simulink model "DemonstratorSimscape"  (R2020b)
settings: Solver=ode113  StartTime=0.0  StopTime=t_stop*0+20  FixedStep=1e-4
values from neighbouring files (symbols this model uses):
  brkD = 0    [main.m]
  brkI = 1e4    (= 10000)    [main.m]
  brkP = 1e5    (= 100000)    [main.m]
  d_drm = 0.5*d_drum    [main.m]
  d_shm = 0.4*d_sheave    [main.m]
  DeltaCable0 = 0    [main.m]
  Droop_scaling = 0    [main.m]
  eta_sh = 0.015    [main.m]
  filt_NUM = ones(1,200)*0.005    [main.m]
  g = 9.80665    [main.m]
  Iw = 0.5*(W.i + M.in*GB.r^2)    [main.m]
  Kp_mul = 0.3    [main.m]
  Lc0 = abs((T.ph-L.height-P.d-L.z0)*0.001)    [main.m]
  Ls1 = ((T.ph-0.5*W.pd)/1000)    [main.m]
  Ls2 = ((0.5*(T.s2+P.d)-2*P.d)/1000)    [main.m]
  M = 50e3    (= 50000)    [calcGrav.m]
  phi0_drm = -90    [main.m]
  phi0_shm = -90    [main.m]
  r_sheave = P.d*0.5    [main.m]
  s = tf('s')    [calcGrav.m]
  tau_brk = 0.001    [main.m]
  tau_em = 60e-3    (= 0.06)    [calcGrav.m]    (also in main.m)
  tau_m = tau_w/GB.r    [main.m]
  Tmax = 400e3    (= 400000)    [main.m]
  Tn_mul = 10    [main.m]
  x_drm = 0.7*r_drum    [main.m]
  x_shm = 0.7*r_sheave    [main.m]
  z0 = 0    [calcGrav.m]    (also in main.m = L.z0-P.d*0.5-P.d-P.d-L.height-T.h1-T.h2-32)
undefined symbols (not defined in the file or in its folder): C, CA, Controller_sampleTime, DiscIntNeverNeededParam, GB, L, P, Part, T, VFD_acceleration_model_factor, VFD_Adapt_factor_lower_p1458, VFD_Adapt_factor_upper_p1459, VFD_Curr_limit_var_p0641, VFD_Current_limit_p0640, VFD_Id_setp_total_r1624, VFD_Iq, VFD_Kp_n_basic_p1460, VFD_M, VFD_M_accel_T_smooth_p1517, VFD_M_lim_var_fixS_src_p1551, VFD_M_max_lower_p1521, VFD_M_max_lower_scal_p1525, VFD_M_max_up_mot_scal_p1524, VFD_M_max_upper_p1520, VFD_n_act_T_smooth_p1442, VFD_n_ctr_Kp_n_up_scal_p1461, VFD_n_ctr_Tn_n_up_sca_p1463, VFD_n_ctrl_adapt_Kp_lower_p1456, VFD_n_ctrl_adapt_Kp_upper_p1457, VFD_n_ctrl_Adpt_sig_Kp_p1455, VFD_n_ctrl_Kp_scal_p1466, VFD_n_ctrl_n_lower_p1464, VFD_n_ctrl_n_upper_p1465, VFD_n_ctrl_Tn_n_lower_p1462, VFD_n_limit_neg_p1086, VFD_n_limit_pos_p1083, VFD_n_limit_setp_p1063, VFD_n_max_p1082, VFD_n_set_filt_1_T_p1416, VFD_P_max_gen_p1531, VFD_P_max_mot_p1530, VFD_PU_I_outp_max_r0289, VFD_RFG_ramp_down_time_p1121, VFD_RFG_ramp_up_time_p1120, VFD_RFG_t_RD_scal_p1139, VFD_RFG_t_RU_scal_p1138, VSD, W, X, Y, Z
libraries: sm_lib x248, nesl_utility x128, simulink x49, pid_lib x4, cstblocks x2, simulink_extras x2
(part 2 of 10)

== system DemonstratorSimscape/EM System/Winch Left (yellow) ==
  theta winch (deg) : Inport
  Rigid Transform : sm_lib/Frames and Transforms/Rigid Transform  TranslationMethod=None  TranslationStandardOffset=0  TranslationLengthUnit=m  TranslationStandardAxis=+Z  TranslationCartesianOffset=[0 0 0]  TranslationROffset=0  TranslationROffsetUnits=m  TranslationZOffset=0  TranslationZOffsetUnits=m  TranslationThetaOffset=0  TranslationThetaOffsetUnits=deg  RotationMethod=StandardAxis  RotationAngleUnits=deg  RotationStandardAxis=+X  RotationAngle=90  RotationArbitraryAxis=[0 0 1]  FollAlignAxisA=+X  BaseAlignAxisA=+Y  FollAlignAxisB=+Y  BaseAlignAxisB=+Z  RotationSequenceAxes=FollowerAxes  RotationSequence=XYX  RotationSequenceAngles=[0 0 0]  RotationSequenceAnglesUnits=deg  RotationMatrix=[1 0 0; 0 1 0; 0 0 1]
  Rigid Transform1 : sm_lib/Frames and Transforms/Rigid Transform  TranslationMethod=StandardAxis  TranslationStandardOffset=1.2*W.w/2  TranslationLengthUnit=mm  TranslationStandardAxis=-Z  TranslationCartesianOffset=[0 0 0]  TranslationROffset=0  TranslationROffsetUnits=m  TranslationZOffset=0  TranslationZOffsetUnits=m  TranslationThetaOffset=0  TranslationThetaOffsetUnits=deg  RotationMethod=None  RotationAngleUnits=deg  RotationStandardAxis=+Z  RotationAngle=0.0  RotationArbitraryAxis=[0 0 1]  FollAlignAxisA=+X  BaseAlignAxisA=+Y  FollAlignAxisB=+Y  BaseAlignAxisB=+Z  RotationSequenceAxes=FollowerAxes  RotationSequence=XYX  RotationSequenceAngles=[0 0 0]  RotationSequenceAnglesUnits=deg  RotationMatrix=[1 0 0; 0 1 0; 0 0 1]
  Rigid Transform2 : sm_lib/Frames and Transforms/Rigid Transform  TranslationMethod=None  TranslationStandardOffset=0  TranslationLengthUnit=m  TranslationStandardAxis=+Z  TranslationCartesianOffset=[0 0 0]  TranslationROffset=0  TranslationROffsetUnits=m  TranslationZOffset=0  TranslationZOffsetUnits=m  TranslationThetaOffset=0  TranslationThetaOffsetUnits=deg  RotationMethod=StandardAxis  RotationAngleUnits=deg  RotationStandardAxis=+Z  RotationAngle=0  RotationArbitraryAxis=[0 0 1]  FollAlignAxisA=+X  BaseAlignAxisA=+Y  FollAlignAxisB=+Y  BaseAlignAxisB=+Z  RotationSequenceAxes=FollowerAxes  RotationSequence=XYX  RotationSequenceAngles=[0 0 0]  RotationSequenceAnglesUnits=deg  RotationMatrix=[1 0 0; 0 1 0; 0 0 1]
  Transform Winch Axis1 : sm_lib/Frames and Transforms/Rigid Transform  TranslationMethod=None  TranslationStandardOffset=0  TranslationLengthUnit=m  TranslationStandardAxis=+Z  TranslationCartesianOffset=[0 0 0]  TranslationROffset=0  TranslationROffsetUnits=m  TranslationZOffset=0  TranslationZOffsetUnits=m  TranslationThetaOffset=0  TranslationThetaOffsetUnits=deg  RotationMethod=StandardAxis  RotationAngleUnits=deg  RotationStandardAxis=+Y  RotationAngle=180  RotationArbitraryAxis=[0 0 1]  FollAlignAxisA=+X  BaseAlignAxisA=+Y  FollAlignAxisB=+Y  BaseAlignAxisB=+Z  RotationSequenceAxes=FollowerAxes  RotationSequence=XYX  RotationSequenceAngles=[0 0 0]  RotationSequenceAnglesUnits=deg  RotationMatrix=[1 0 0; 0 1 0; 0 0 1]
  Variable Winch Inertia : Subsystem
  Winch1 : sm_lib/Body Elements/Cylindrical Solid  GraphicAmbientColor=[0.15 0.15 0.15 1.0]  BasedOnType=Mass  CenterOfMass=[0 0 W.w*0.5]  CenterOfMassUnits=m  GraphicDiffuseColor=[1.0 1.0 1.0]  CylinderLength=W.w  CylinderLengthUnits=mm  CylinderRadius=W.d*0.5  CylinderRadiusUnits=mm  Density=0  DensityUnits=kg/m^3  DoExposeReferenceFrame=off  GraphicEmissiveColor=[0.0 0.0 0.0 1.0]  ExportEntireGeometry=off  SerializedFrames=<Frames><Frame><Id>Frame1</Id><Value><Name>F1</Name><Origin><Source>ReferenceFrame</Source><FeatureName></FeatureName></Origin><PrimaryAxis><DefinedDirection>+Z</DefinedDirection><Source>ReferenceFrame</Source><SourceDirection>-Y</SourceDirection><FeatureName></FeatureName></PrimaryAxis><SecondaryAxis><DefinedDirection>+X</DefinedDirection><Source>ReferenceFrame</Source><SourceDirection>+X</SourceDirection><FeatureName></FeatureName></SecondaryAxis></Value></Frame></Frames>  MarkerShape=Frame  MarkerSize=10  GraphicType=FromGeometry  InertiaType=CalculateFromGeometry  Mass=W.mass  MassUnits=kg  MomentsOfInertia=[1 1 1]*Iw  MomentsOfInertiaUnits=kg*m^2  GraphicOpacity=1.0  ProductsOfInertia=[0 0 0]  ProductsOfInertiaUnits=kg*m^2  GraphicShininess=10  GraphicSpecularColor=[0.8 0.8 0.8]  GraphicVisPropType=SimpleVisualProperties
  tags : Subsystem  mask{phi0=phi0_drm, s=1}
      mask prompts: phi0 "angle (deg)"; s "direction (1 | -1)"
  W : PMIOPort  Side=Right
  F : PMIOPort  Port=2  Side=Left
  r_winch (mm) : Outport  VectorParamsAs1DForOutWhenUnconnected=off
  wires:
  theta winch (deg)/1 -> Variable Winch Inertia/1(WinchAngle (deg))
  Variable Winch Inertia/2(WinchRadius (mm)) -> r_winch (mm)/1
  connections:
  W/RConn1 -- Rigid Transform2/RConn1 -- Transform Winch Axis1/RConn1
  Winch1/LConn1 -- Rigid Transform/LConn1 -- Variable Winch Inertia/RConn1
  Rigid Transform/RConn1 -- Rigid Transform2/LConn1
  Transform Winch Axis1/LConn1 -- Rigid Transform1/LConn1 -- F/RConn1
  tags/LConn1 -- Rigid Transform1/RConn1

== system DemonstratorSimscape/EM System/Winch Right (blue) ==
  theta winch (deg) : Inport
  Rigid Transform : sm_lib/Frames and Transforms/Rigid Transform  TranslationMethod=None  TranslationStandardOffset=0  TranslationLengthUnit=m  TranslationStandardAxis=+Z  TranslationCartesianOffset=[0 0 0]  TranslationROffset=0  TranslationROffsetUnits=m  TranslationZOffset=0  TranslationZOffsetUnits=m  TranslationThetaOffset=0  TranslationThetaOffsetUnits=deg  RotationMethod=StandardAxis  RotationAngleUnits=deg  RotationStandardAxis=+X  RotationAngle=90  RotationArbitraryAxis=[0 0 1]  FollAlignAxisA=+X  BaseAlignAxisA=+Y  FollAlignAxisB=+Y  BaseAlignAxisB=+Z  RotationSequenceAxes=FollowerAxes  RotationSequence=XYX  RotationSequenceAngles=[0 0 0]  RotationSequenceAnglesUnits=deg  RotationMatrix=[1 0 0; 0 1 0; 0 0 1]
  Rigid Transform1 : sm_lib/Frames and Transforms/Rigid Transform  TranslationMethod=StandardAxis  TranslationStandardOffset=1.05*W.w/2  TranslationLengthUnit=mm  TranslationStandardAxis=+Z  TranslationCartesianOffset=[0 0 0]  TranslationROffset=0  TranslationROffsetUnits=m  TranslationZOffset=0  TranslationZOffsetUnits=m  TranslationThetaOffset=0  TranslationThetaOffsetUnits=deg  RotationMethod=None  RotationAngleUnits=deg  RotationStandardAxis=+Z  RotationAngle=0.0  RotationArbitraryAxis=[0 0 1]  FollAlignAxisA=+X  BaseAlignAxisA=+Y  FollAlignAxisB=+Y  BaseAlignAxisB=+Z  RotationSequenceAxes=FollowerAxes  RotationSequence=XYX  RotationSequenceAngles=[0 0 0]  RotationSequenceAnglesUnits=deg  RotationMatrix=[1 0 0; 0 1 0; 0 0 1]
  Variable Winch Inertia : Subsystem
  Winch2 : sm_lib/Body Elements/Cylindrical Solid  GraphicAmbientColor=[0.15 0.15 0.15 1.0]  BasedOnType=Mass  CenterOfMass=[0 0 W.w*0.5]  CenterOfMassUnits=m  GraphicDiffuseColor=[1.0 1.0 1.0]  CylinderLength=W.w  CylinderLengthUnits=mm  CylinderRadius=W.d*0.5  CylinderRadiusUnits=mm  Density=0  DensityUnits=kg/m^3  DoExposeReferenceFrame=off  GraphicEmissiveColor=[0.0 0.0 0.0 1.0]  ExportEntireGeometry=off  SerializedFrames=<Frames><Frame><Id>Frame1</Id><Value><Name>F1</Name><Origin><Source>ReferenceFrame</Source><FeatureName></FeatureName></Origin><PrimaryAxis><DefinedDirection>+Z</DefinedDirection><Source>ReferenceFrame</Source><SourceDirection>-Y</SourceDirection><FeatureName></FeatureName></PrimaryAxis><SecondaryAxis><DefinedDirection>+X</DefinedDirection><Source>ReferenceFrame</Source><SourceDirection>+X</SourceDirection><FeatureName></FeatureName></SecondaryAxis></Value></Frame></Frames>  MarkerShape=Frame  MarkerSize=10  GraphicType=FromGeometry  InertiaType=CalculateFromGeometry  Mass=W.mass  MassUnits=kg  MomentsOfInertia=[1 1 1]*Iw  MomentsOfInertiaUnits=kg*m^2  GraphicOpacity=1.0  ProductsOfInertia=[0 0 0]  ProductsOfInertiaUnits=kg*m^2  GraphicShininess=10  GraphicSpecularColor=[0.8 0.8 0.8]  GraphicVisPropType=SimpleVisualProperties
  tags : Subsystem  mask{phi0=phi0_drm, s=1}
      mask prompts: phi0 "angle (deg)"; s "direction (1 | -1)"
  W : PMIOPort  Side=Right
  F : PMIOPort  Port=2  Side=Left
  r_winch (mm) : Outport  VectorParamsAs1DForOutWhenUnconnected=off
  wires:
  theta winch (deg)/1 -> Variable Winch Inertia/1(WinchAngle (deg))
  Variable Winch Inertia/2(WinchRadius (mm)) -> r_winch (mm)/1
  connections:
  F/RConn1 -- Rigid Transform1/LConn1 -- Rigid Transform/RConn1 -- W/RConn1
  Winch2/LConn1 -- Variable Winch Inertia/RConn1 -- Rigid Transform/LConn1
  tags/LConn1 -- Rigid Transform1/RConn1

== system DemonstratorSimscape/Transmission System/Anchor and Load ==
  w7 : Inport
  w6 : Inport  Port=2
  w4 : Inport  Port=3
  w2 : Inport  Port=4
  w1 : Inport  Port=5
  wL : Inport  Port=6
  wR : Inport  Port=7
  Alg Loop Break : Memory
  CableFlex_Left : Subsystem
  CableFlex_Right : Subsystem
  CableRigid_Left : Subsystem  Commented=on
  CableRigid_Right : Subsystem  Commented=on
  FlexDisp_Left : Subsystem
  FlexDisp_Right : Subsystem
  Load : Subsystem
  Sheave_03 : Subsystem
  Sheave_05 : Subsystem
  cable mass : Subsystem
  Conn56 : PMIOPort  Side=Left
  ConnCentre : PMIOPort  Port=2  Side=Left
  Conn34 : PMIOPort  Port=3  Side=Left
  Conn54 : PMIOPort  Port=4  Side=Left
  Conn32 : PMIOPort  Port=5  Side=Left
  LoadPos (mm) : Outport  VectorParamsAs1DForOutWhenUnconnected=off
  LoadVel (m/s) : Outport  Port=2  VectorParamsAs1DForOutWhenUnconnected=off
  tag scope: CableMass=global, NetCableMass=global
  wires:
  w4/1 -> FlexDisp_Right/1(w4), FlexDisp_Left/4(w4)
  Alg Loop Break/1 -> FlexDisp_Right/5(LoadAcc), FlexDisp_Left/5(LoadAcc)
  wR/1 -> FlexDisp_Right/4(wR)
  wL/1 -> FlexDisp_Left/1(wL)
  w2/1 -> FlexDisp_Left/3(w2)
  w1/1 -> FlexDisp_Left/2(w1)
  w7/1 -> FlexDisp_Right/3(w7)
  w6/1 -> FlexDisp_Right/2(w6)
  Sheave_03/1(w (rad/s)) -> FlexDisp_Left/6(w3)
  Sheave_05/1(w (rad/s)) -> FlexDisp_Right/6(w5)
  Load/1(LoadAcc (m/s^2)) -> Alg Loop Break/1
  Load/2(LoadPos (mm)) -> cable mass/1("LoadPos [mm] "), LoadPos (mm)/1
  Load/3(LoadVel (m/s)) -> LoadVel (m/s)/1
  cable mass/1(net cable mass [kg]) -> [NetCableMass], Load/1(CableMass (kg))
  cable mass/3(cable mass [kg]) -> [CableMass]
  FlexDisp_Left/1(disp (m)) -> CableFlex_Left/1(disp [m])
  FlexDisp_Right/1(disp (m)) -> CableFlex_Right/1(disp [m])
  connections:
  Conn34/RConn1 -- Sheave_03/LConn1
  Conn32/RConn1 -- Sheave_03/LConn2
  Sheave_05/LConn1 -- Conn56/RConn1
  Conn54/RConn1 -- Sheave_05/LConn2
  Sheave_03/RConn1 -- CableRigid_Left/LConn1 -- CableFlex_Left/LConn1
  CableFlex_Right/LConn1 -- CableRigid_Right/LConn1 -- Sheave_05/RConn1
  CableFlex_Left/RConn1 -- CableRigid_Left/RConn1 -- Load/LConn1
  Load/RConn1 -- ConnCentre/RConn1
  CableFlex_Right/RConn1 -- CableRigid_Right/RConn1 -- Load/LConn2

== system DemonstratorSimscape/Transmission System/Roof Pulley Set ==
  Cable Winch : sm_lib/Belts and Cables/Belt-Cable Properties  Commented=on  DrumBeltCableAlignment=MonitoredPlanar  GraphicType=PitchLine  GraphicVisPropType=SimpleVisualProperties  GraphicDiffuseColor=[0.9 0.35 0]  GraphicSpecularColor=[0.5 0.5 0.5 1.0]  GraphicAmbientColor=[0.15 0.15 0.15 1.0]  GraphicEmissiveColor=[0.0 0.0 0.0 1.0]  GraphicShininess=75  GraphicOpacity=1
      settings: SourceProductBaseCode=MS
  Cable Winch1 : sm_lib/Belts and Cables/Belt-Cable Properties  DrumBeltCableAlignment=MonitoredPlanar  GraphicType=PitchLine  GraphicVisPropType=SimpleVisualProperties  GraphicDiffuseColor=[0.9 0.35 0]  GraphicSpecularColor=[0.5 0.5 0.5 1.0]  GraphicAmbientColor=[0.15 0.15 0.15 1.0]  GraphicEmissiveColor=[0.0 0.0 0.0 1.0]  GraphicShininess=75  GraphicOpacity=1
      settings: SourceProductBaseCode=MS
  ENDS : Subsystem  Commented=on
  Rigid Transform1 : sm_lib/Frames and Transforms/Rigid Transform  TranslationMethod=Cartesian  TranslationStandardOffset=0  TranslationLengthUnit=mm  TranslationStandardAxis=+Z  TranslationCartesianOffset="[1.5*P.d+0.5*P.Bd  P.up 0]"  TranslationROffset=0  TranslationROffsetUnits=m  TranslationZOffset=0  TranslationZOffsetUnits=m  TranslationThetaOffset=0  TranslationThetaOffsetUnits=deg  RotationMethod=None  RotationAngleUnits=deg  RotationStandardAxis=+Z  RotationAngle=0.0  RotationArbitraryAxis=[0 0 1]  FollAlignAxisA=+X  BaseAlignAxisA=+Y  FollAlignAxisB=+Y  BaseAlignAxisB=+Z  RotationSequenceAxes=FollowerAxes  RotationSequence=XYX  RotationSequenceAngles=[0 0 0]  RotationSequenceAnglesUnits=deg  RotationMatrix=[1 0 0; 0 1 0; 0 0 1]
  Rigid Transform2 : sm_lib/Frames and Transforms/Rigid Transform  TranslationMethod=Cartesian  TranslationStandardOffset=0  TranslationLengthUnit=mm  TranslationStandardAxis=+Z  TranslationCartesianOffset="[-1.5*P.d-0.5*P.Bd  P.up 0]"  TranslationROffset=0  TranslationROffsetUnits=m  TranslationZOffset=0  TranslationZOffsetUnits=m  TranslationThetaOffset=0  TranslationThetaOffsetUnits=deg  RotationMethod=None  RotationAngleUnits=deg  RotationStandardAxis=+Z  RotationAngle=0.0  RotationArbitraryAxis=[0 0 1]  FollAlignAxisA=+X  BaseAlignAxisA=+Y  FollAlignAxisB=+Y  BaseAlignAxisB=+Z  RotationSequenceAxes=FollowerAxes  RotationSequence=XYX  RotationSequenceAngles=[0 0 0]  RotationSequenceAnglesUnits=deg  RotationMatrix=[1 0 0; 0 1 0; 0 0 1]
  Rigid Transform20 : sm_lib/Frames and Transforms/Rigid Transform  TranslationMethod=Cartesian  TranslationStandardOffset=0  TranslationLengthUnit=mm  TranslationStandardAxis=+Z  TranslationCartesianOffset="[-0.5*T.s2+0.5*P.d  P.up 0]"  TranslationROffset=0  TranslationROffsetUnits=m  TranslationZOffset=0  TranslationZOffsetUnits=m  TranslationThetaOffset=0  TranslationThetaOffsetUnits=deg  RotationMethod=None  RotationAngleUnits=deg  RotationStandardAxis=+Z  RotationAngle=0.0  RotationArbitraryAxis=[0 0 1]  FollAlignAxisA=+X  BaseAlignAxisA=+Y  FollAlignAxisB=+Y  BaseAlignAxisB=+Z  RotationSequenceAxes=FollowerAxes  RotationSequence=XYX  RotationSequenceAngles=[0 0 0]  RotationSequenceAnglesUnits=deg  RotationMatrix=[1 0 0; 0 1 0; 0 0 1]
  Rigid Transform3 : sm_lib/Frames and Transforms/Rigid Transform  TranslationMethod=Cartesian  TranslationStandardOffset=0  TranslationLengthUnit=mm  TranslationStandardAxis=+Z  TranslationCartesianOffset="[0  P.up 0]"  TranslationROffset=0  TranslationROffsetUnits=m  TranslationZOffset=0  TranslationZOffsetUnits=m  TranslationThetaOffset=0  TranslationThetaOffsetUnits=deg  RotationMethod=None  RotationAngleUnits=deg  RotationStandardAxis=+Z  RotationAngle=0.0  RotationArbitraryAxis=[0 0 1]  FollAlignAxisA=+X  BaseAlignAxisA=+Y  FollAlignAxisB=+Y  BaseAlignAxisB=+Z  RotationSequenceAxes=FollowerAxes  RotationSequence=XYX  RotationSequenceAngles=[0 0 0]  RotationSequenceAnglesUnits=deg  RotationMatrix=[1 0 0; 0 1 0; 0 0 1]
  Rigid Transform4 : sm_lib/Frames and Transforms/Rigid Transform  TranslationMethod=Cartesian  TranslationStandardOffset=0  TranslationLengthUnit=mm  TranslationStandardAxis=+Z  TranslationCartesianOffset="[0.5*T.s2-0.5*P.d  P.up 0]"  TranslationROffset=0  TranslationROffsetUnits=m  TranslationZOffset=0  TranslationZOffsetUnits=m  TranslationThetaOffset=0  TranslationThetaOffsetUnits=deg  RotationMethod=None  RotationAngleUnits=deg  RotationStandardAxis=+Z  RotationAngle=0.0  RotationArbitraryAxis=[0 0 1]  FollAlignAxisA=+X  BaseAlignAxisA=+Y  FollAlignAxisB=+Y  BaseAlignAxisB=+Z  RotationSequenceAxes=FollowerAxes  RotationSequence=XYX  RotationSequenceAngles=[0 0 0]  RotationSequenceAnglesUnits=deg  RotationMatrix=[1 0 0; 0 1 0; 0 0 1]
  Sheave_01 : Subsystem
  Sheave_02 : Subsystem
  Sheave_04 : Subsystem
  Sheave_06 : Subsystem
  Sheave_07 : Subsystem
  ConnS65 : PMIOPort  Side=Right
  ConnEndL : PMIOPort  Port=2  Side=Right
  World : PMIOPort  Port=3  Side=Left
  ConnEndR : PMIOPort  Port=4  Side=Right
  ConnCentre : PMIOPort  Port=5  Side=Right
  ConnS23 : PMIOPort  Port=6  Side=Right
  RWinch : PMIOPort  Port=7  Side=Left
  LWinch : PMIOPort  Port=8  Side=Left
  w7 : Outport  VectorParamsAs1DForOutWhenUnconnected=off
  w6 : Outport  Port=2  VectorParamsAs1DForOutWhenUnconnected=off
  w4 : Outport  Port=3  VectorParamsAs1DForOutWhenUnconnected=off
  w2 : Outport  Port=4  VectorParamsAs1DForOutWhenUnconnected=off
  w1 : Outport  Port=5  VectorParamsAs1DForOutWhenUnconnected=off
  wires:
  Sheave_04/1(w5) -> w4/1
  Sheave_01/1(w (rad/s)) -> w1/1
  Sheave_02/1(w (rad/s)) -> w2/1
  Sheave_06/1(w (rad/s)) -> w6/1
  Sheave_07/1(w (rad/s)) -> w7/1
  connections:
  Cable Winch/LConn1 -- ENDS/RConn1 -- Sheave_04/RConn1 -- ConnEndL/RConn1
  ConnEndR/RConn1 -- Cable Winch1/LConn1 -- Sheave_04/RConn2 -- ENDS/RConn2
  ENDS/LConn1 -- ConnCentre/RConn1 -- Rigid Transform3/RConn1 -- Sheave_04/LConn1
  World/RConn1 -- Rigid Transform20/LConn1 -- Rigid Transform2/LConn1 -- Rigid Transform3/LConn1 -- Rigid Transform1/LConn1 -- Rigid Transform4/LConn1
  Rigid Transform20/RConn1 -- Sheave_01/LConn1
  Sheave_01/RConn2 -- LWinch/RConn1
  Sheave_02/LConn1 -- Rigid Transform2/RConn1
  Sheave_02/RConn1 -- ConnS23/RConn1
  Sheave_01/RConn1 -- Sheave_02/RConn2
  Sheave_06/LConn1 -- Rigid Transform1/RConn1
  ConnS65/RConn1 -- Sheave_06/RConn2
  Rigid Transform4/RConn1 -- Sheave_07/LConn1
  Sheave_07/RConn1 -- RWinch/RConn1
  Sheave_06/RConn1 -- Sheave_07/RConn2

== system DemonstratorSimscape/Transmission System/Tower structure ==
  Rigid Transform10 : sm_lib/Frames and Transforms/Rigid Transform  TranslationMethod=Cartesian  TranslationStandardOffset=0  TranslationLengthUnit=mm  TranslationStandardAxis=+Z  TranslationCartesianOffset=[0 -(T.rs+T.h2)*.5 T.h0+T.hl1+T.hl2*.5]  TranslationROffset=0  TranslationROffsetUnits=m  TranslationZOffset=0  TranslationZOffsetUnits=m  TranslationThetaOffset=0  TranslationThetaOffsetUnits=deg  RotationMethod=None  RotationAngleUnits=deg  RotationStandardAxis=+Z  RotationAngle=0.0  RotationArbitraryAxis=[0 0 1]  FollAlignAxisA=+X  BaseAlignAxisA=+Y  FollAlignAxisB=+Y  BaseAlignAxisB=+Z  RotationSequenceAxes=FollowerAxes  RotationSequence=XYX  RotationSequenceAngles=[0 0 0]  RotationSequenceAnglesUnits=deg  RotationMatrix=[1 0 0; 0 1 0; 0 0 1]
  Rigid Transform11 : sm_lib/Frames and Transforms/Rigid Transform  TranslationMethod=Cartesian  TranslationStandardOffset=0  TranslationLengthUnit=mm  TranslationStandardAxis=+Z  TranslationCartesianOffset=[ -(T.s*.5+T.c)*.5 0 T.h0+T.hl1*.5]  TranslationROffset=0  TranslationROffsetUnits=m  TranslationZOffset=0  TranslationZOffsetUnits=m  TranslationThetaOffset=0  TranslationThetaOffsetUnits=deg  RotationMethod=None  RotationAngleUnits=deg  RotationStandardAxis=+Z  RotationAngle=0.0  RotationArbitraryAxis=[0 0 1]  FollAlignAxisA=+X  BaseAlignAxisA=+Y  FollAlignAxisB=+Y  BaseAlignAxisB=+Z  RotationSequenceAxes=FollowerAxes  RotationSequence=XYX  RotationSequenceAngles=[0 0 0]  RotationSequenceAnglesUnits=deg  RotationMatrix=[1 0 0; 0 1 0; 0 0 1]
  Rigid Transform12 : sm_lib/Frames and Transforms/Rigid Transform  TranslationMethod=Cartesian  TranslationStandardOffset=0  TranslationLengthUnit=mm  TranslationStandardAxis=+Z  TranslationCartesianOffset=[ (T.s*.5+T.c)*.5 0 T.h0+T.hl1*.5]  TranslationROffset=0  TranslationROffsetUnits=m  TranslationZOffset=0  TranslationZOffsetUnits=m  TranslationThetaOffset=0  TranslationThetaOffsetUnits=deg  RotationMethod=None  RotationAngleUnits=deg  RotationStandardAxis=+Z  RotationAngle=0.0  RotationArbitraryAxis=[0 0 1]  FollAlignAxisA=+X  BaseAlignAxisA=+Y  FollAlignAxisB=+Y  BaseAlignAxisB=+Z  RotationSequenceAxes=FollowerAxes  RotationSequence=XYX  RotationSequenceAngles=[0 0 0]  RotationSequenceAnglesUnits=deg  RotationMatrix=[1 0 0; 0 1 0; 0 0 1]
  Rigid Transform13 : sm_lib/Frames and Transforms/Rigid Transform  TranslationMethod=None  TranslationStandardOffset=0  TranslationLengthUnit=m  TranslationStandardAxis=+Z  TranslationCartesianOffset=[0 0 0]  TranslationROffset=0  TranslationROffsetUnits=m  TranslationZOffset=0  TranslationZOffsetUnits=m  TranslationThetaOffset=0  TranslationThetaOffsetUnits=deg  RotationMethod=StandardAxis  RotationAngleUnits=deg  RotationStandardAxis=+X  RotationAngle=-90  RotationArbitraryAxis=[0 0 1]  FollAlignAxisA=+X  BaseAlignAxisA=+Y  FollAlignAxisB=+Y  BaseAlignAxisB=+Z  RotationSequenceAxes=FollowerAxes  RotationSequence=XYX  RotationSequenceAngles=[0 0 0]  RotationSequenceAnglesUnits=deg  RotationMatrix=[1 0 0; 0 1 0; 0 0 1]
  Rigid Transform14 : sm_lib/Frames and Transforms/Rigid Transform  TranslationMethod=Cartesian  TranslationStandardOffset=0  TranslationLengthUnit=mm  TranslationStandardAxis=+Z  TranslationCartesianOffset=[-0.5*(T.s+T.c) -0.5*(T.s+T.c) T.h0/2]  TranslationROffset=0  TranslationROffsetUnits=m  TranslationZOffset=0  TranslationZOffsetUnits=m  TranslationThetaOffset=0  TranslationThetaOffsetUnits=deg  RotationMethod=None  RotationAngleUnits=deg  RotationStandardAxis=+Z  RotationAngle=0.0  RotationArbitraryAxis=[0 0 1]  FollAlignAxisA=+X  BaseAlignAxisA=+Y  FollAlignAxisB=+Y  BaseAlignAxisB=+Z  RotationSequenceAxes=FollowerAxes  RotationSequence=XYX  RotationSequenceAngles=[0 0 0]  RotationSequenceAnglesUnits=deg  RotationMatrix=[1 0 0; 0 1 0; 0 0 1]
  Rigid Transform15 : sm_lib/Frames and Transforms/Rigid Transform  TranslationMethod=Cartesian  TranslationStandardOffset=0  TranslationLengthUnit=mm  TranslationStandardAxis=+Z  TranslationCartesianOffset=[0 (T.s+T.c)*.5 T.h0+T.hl1*.5]  TranslationROffset=0  TranslationROffsetUnits=m  TranslationZOffset=0  TranslationZOffsetUnits=m  TranslationThetaOffset=0  TranslationThetaOffsetUnits=deg  RotationMethod=None  RotationAngleUnits=deg  RotationStandardAxis=+Z  RotationAngle=0.0  RotationArbitraryAxis=[0 0 1]  FollAlignAxisA=+X  BaseAlignAxisA=+Y  FollAlignAxisB=+Y  BaseAlignAxisB=+Z  RotationSequenceAxes=FollowerAxes  RotationSequence=XYX  RotationSequenceAngles=[0 0 0]  RotationSequenceAnglesUnits=deg  RotationMatrix=[1 0 0; 0 1 0; 0 0 1]
  Rigid Transform16 : sm_lib/Frames and Transforms/Rigid Transform  TranslationMethod=Cartesian  TranslationStandardOffset=0  TranslationLengthUnit=mm  TranslationStandardAxis=+Z  TranslationCartesianOffset=[0 -(T.s+T.c)*.5 T.h0+T.hl1*.5]  TranslationROffset=0  TranslationROffsetUnits=m  TranslationZOffset=0  TranslationZOffsetUnits=m  TranslationThetaOffset=0  TranslationThetaOffsetUnits=deg  RotationMethod=None  RotationAngleUnits=deg  RotationStandardAxis=+Z  RotationAngle=0.0  RotationArbitraryAxis=[0 0 1]  FollAlignAxisA=+X  BaseAlignAxisA=+Y  FollAlignAxisB=+Y  BaseAlignAxisB=+Z  RotationSequenceAxes=FollowerAxes  RotationSequence=XYX  RotationSequenceAngles=[0 0 0]  RotationSequenceAnglesUnits=deg  RotationMatrix=[1 0 0; 0 1 0; 0 0 1]
  Rigid Transform17 : sm_lib/Frames and Transforms/Rigid Transform  TranslationMethod=Cartesian  TranslationStandardOffset=0  TranslationLengthUnit=mm  TranslationStandardAxis=+Z  TranslationCartesianOffset=[ -(T.s+T.c)*.5 0 T.h0+T.hl1*.5]  TranslationROffset=0  TranslationROffsetUnits=m  TranslationZOffset=0  TranslationZOffsetUnits=m  TranslationThetaOffset=0  TranslationThetaOffsetUnits=deg  RotationMethod=None  RotationAngleUnits=deg  RotationStandardAxis=+Z  RotationAngle=0.0  RotationArbitraryAxis=[0 0 1]  FollAlignAxisA=+X  BaseAlignAxisA=+Y  FollAlignAxisB=+Y  BaseAlignAxisB=+Z  RotationSequenceAxes=FollowerAxes  RotationSequence=XYX  RotationSequenceAngles=[0 0 0]  RotationSequenceAnglesUnits=deg  RotationMatrix=[1 0 0; 0 1 0; 0 0 1]
  Rigid Transform18 : sm_lib/Frames and Transforms/Rigid Transform  TranslationMethod=Cartesian  TranslationStandardOffset=0  TranslationLengthUnit=mm  TranslationStandardAxis=+Z  TranslationCartesianOffset=[ (T.s+T.c)*.5 0 T.h0+T.hl1*.5]  TranslationROffset=0  TranslationROffsetUnits=m  TranslationZOffset=0  TranslationZOffsetUnits=m  TranslationThetaOffset=0  TranslationThetaOffsetUnits=deg  RotationMethod=None  RotationAngleUnits=deg  RotationStandardAxis=+Z  RotationAngle=0.0  RotationArbitraryAxis=[0 0 1]  FollAlignAxisA=+X  BaseAlignAxisA=+Y  FollAlignAxisB=+Y  BaseAlignAxisB=+Z  RotationSequenceAxes=FollowerAxes  RotationSequence=XYX  RotationSequenceAngles=[0 0 0]  RotationSequenceAnglesUnits=deg  RotationMatrix=[1 0 0; 0 1 0; 0 0 1]
  Rigid Transform19 : sm_lib/Frames and Transforms/Rigid Transform  TranslationMethod=Cartesian  TranslationStandardOffset=0  TranslationLengthUnit=mm  TranslationStandardAxis=+Z  TranslationCartesianOffset=[0 (T.rs+T.h2)*.5 T.h0+T.hl1+T.hl2*.5]  TranslationROffset=0  TranslationROffsetUnits=m  TranslationZOffset=0  TranslationZOffsetUnits=m  TranslationThetaOffset=0  TranslationThetaOffsetUnits=deg  RotationMethod=None  RotationAngleUnits=deg  RotationStandardAxis=+Z  RotationAngle=0.0  RotationArbitraryAxis=[0 0 1]  FollAlignAxisA=+X  BaseAlignAxisA=+Y  FollAlignAxisB=+Y  BaseAlignAxisB=+Z  RotationSequenceAxes=FollowerAxes  RotationSequence=XYX  RotationSequenceAngles=[0 0 0]  RotationSequenceAnglesUnits=deg  RotationMatrix=[1 0 0; 0 1 0; 0 0 1]
  Rigid Transform6 : sm_lib/Frames and Transforms/Rigid Transform  TranslationMethod=Cartesian  TranslationStandardOffset=0  TranslationLengthUnit=mm  TranslationStandardAxis=+Z  TranslationCartesianOffset=[0 0 -T.bh/2]  TranslationROffset=0  TranslationROffsetUnits=m  TranslationZOffset=0  TranslationZOffsetUnits=m  TranslationThetaOffset=0  TranslationThetaOffsetUnits=deg  RotationMethod=None  RotationAngleUnits=deg  RotationStandardAxis=+Z  RotationAngle=0.0  RotationArbitraryAxis=[0 0 1]  FollAlignAxisA=+X  BaseAlignAxisA=+Y  FollAlignAxisB=+Y  BaseAlignAxisB=+Z  RotationSequenceAxes=FollowerAxes  RotationSequence=XYX  RotationSequenceAngles=[0 0 0]  RotationSequenceAnglesUnits=deg  RotationMatrix=[1 0 0; 0 1 0; 0 0 1]
  Rigid Transform7 : sm_lib/Frames and Transforms/Rigid Transform  TranslationMethod=Cartesian  TranslationStandardOffset=0  TranslationLengthUnit=mm  TranslationStandardAxis=+Z  TranslationCartesianOffset=[0.5*(T.s+T.c) 0.5*(T.s+T.c) T.h0/2]  TranslationROffset=0  TranslationROffsetUnits=m  TranslationZOffset=0  TranslationZOffsetUnits=m  TranslationThetaOffset=0  TranslationThetaOffsetUnits=deg  RotationMethod=None  RotationAngleUnits=deg  RotationStandardAxis=+Z  RotationAngle=0.0  RotationArbitraryAxis=[0 0 1]  FollAlignAxisA=+X  BaseAlignAxisA=+Y  FollAlignAxisB=+Y  BaseAlignAxisB=+Z  RotationSequenceAxes=FollowerAxes  RotationSequence=XYX  RotationSequenceAngles=[0 0 0]  RotationSequenceAnglesUnits=deg  RotationMatrix=[1 0 0; 0 1 0; 0 0 1]
  Rigid Transform8 : sm_lib/Frames and Transforms/Rigid Transform  TranslationMethod=Cartesian  TranslationStandardOffset=0  TranslationLengthUnit=mm  TranslationStandardAxis=+Z  TranslationCartesianOffset=[-0.5*(T.s+T.c) 0.5*(T.s+T.c) T.h0/2]  TranslationROffset=0  TranslationROffsetUnits=m  TranslationZOffset=0  TranslationZOffsetUnits=m  TranslationThetaOffset=0  TranslationThetaOffsetUnits=deg  RotationMethod=None  RotationAngleUnits=deg  RotationStandardAxis=+Z  RotationAngle=0.0  RotationArbitraryAxis=[0 0 1]  FollAlignAxisA=+X  BaseAlignAxisA=+Y  FollAlignAxisB=+Y  BaseAlignAxisB=+Z  RotationSequenceAxes=FollowerAxes  RotationSequence=XYX  RotationSequenceAngles=[0 0 0]  RotationSequenceAnglesUnits=deg  RotationMatrix=[1 0 0; 0 1 0; 0 0 1]
  Rigid Transform9 : sm_lib/Frames and Transforms/Rigid Transform  TranslationMethod=Cartesian  TranslationStandardOffset=0  TranslationLengthUnit=mm  TranslationStandardAxis=+Z  TranslationCartesianOffset=[0.5*(T.s+T.c) -0.5*(T.s+T.c) T.h0/2]  TranslationROffset=0  TranslationROffsetUnits=m  TranslationZOffset=0  TranslationZOffsetUnits=m  TranslationThetaOffset=0  TranslationThetaOffsetUnits=deg  RotationMethod=None  RotationAngleUnits=deg  RotationStandardAxis=+Z  RotationAngle=0.0  RotationArbitraryAxis=[0 0 1]  FollAlignAxisA=+X  BaseAlignAxisA=+Y  FollAlignAxisB=+Y  BaseAlignAxisB=+Z  RotationSequenceAxes=FollowerAxes  RotationSequence=XYX  RotationSequenceAngles=[0 0 0]  RotationSequenceAnglesUnits=deg  RotationMatrix=[1 0 0; 0 1 0; 0 0 1]
  Tower base : sm_lib/Body Elements/Brick Solid  GraphicAmbientColor=[0.15 0.15 0.15 1.0]  BasedOnType=Density  BrickDimensions=[T.b T.b T.bh]  BrickDimensionUnits=mm  CenterOfMass=[0 0 0]  CenterOfMassUnits=m  GraphicDiffuseColor=[0.5 0.5 0.5]  Density=500000000000000000000000  DensityUnits=kg/m^3  DoExposeReferenceFrame=on  GraphicEmissiveColor=[0.0 0.0 0.0 1.0]  ExportEntireGeometry=off  SerializedFrames=<Frames/>  MarkerShape=Sphere  MarkerSize=10  GraphicType=FromGeometry  InertiaType=CalculateFromGeometry  Mass=1  MassUnits=kg  MomentsOfInertia=[1 1 1]  MomentsOfInertiaUnits=kg*m^2  GraphicOpacity=0.5  ProductsOfInertia=[0 0 0]  ProductsOfInertiaUnits=kg*m^2  GraphicShininess=75  GraphicSpecularColor=[0.5 0.5 0.5 1.0]  GraphicVisPropType=SimpleVisualProperties
  Tower column 1 : sm_lib/Body Elements/Brick Solid  GraphicAmbientColor=[0.15 0.15 0.15 1.0]  BasedOnType=Density  BrickDimensions=[T.c T.c T.h0]  BrickDimensionUnits=mm  CenterOfMass=[0 0 0]  CenterOfMassUnits=m  GraphicDiffuseColor=[0.8 0.0 0.2]  Density=1000  DensityUnits=kg/m^3  DoExposeReferenceFrame=on  GraphicEmissiveColor=[0.0 0.0 0.0 1.0]  ExportEntireGeometry=off  SerializedFrames=<Frames/>  MarkerShape=Sphere  MarkerSize=10  GraphicType=FromGeometry  InertiaType=CalculateFromGeometry  Mass=1  MassUnits=kg  MomentsOfInertia=[1 1 1]  MomentsOfInertiaUnits=kg*m^2  GraphicOpacity=1.0  ProductsOfInertia=[0 0 0]  ProductsOfInertiaUnits=kg*m^2  GraphicShininess=75  GraphicSpecularColor=[0.5 0.5 0.5 1.0]  GraphicVisPropType=SimpleVisualProperties
  Tower column 2 : sm_lib/Body Elements/Brick Solid  GraphicAmbientColor=[0.15 0.15 0.15 1.0]  BasedOnType=Density  BrickDimensions=[T.c T.c T.h0]  BrickDimensionUnits=mm  CenterOfMass=[0 0 0]  CenterOfMassUnits=m  GraphicDiffuseColor=[0.8 0.0 0.2]  Density=1000  DensityUnits=kg/m^3  DoExposeReferenceFrame=on  GraphicEmissiveColor=[0.0 0.0 0.0 1.0]  ExportEntireGeometry=off  SerializedFrames=<Frames/>  MarkerShape=Sphere  MarkerSize=10  GraphicType=FromGeometry  InertiaType=CalculateFromGeometry  Mass=1  MassUnits=kg  MomentsOfInertia=[1 1 1]  MomentsOfInertiaUnits=kg*m^2  GraphicOpacity=1.0  ProductsOfInertia=[0 0 0]  ProductsOfInertiaUnits=kg*m^2  GraphicShininess=75  GraphicSpecularColor=[0.5 0.5 0.5 1.0]  GraphicVisPropType=SimpleVisualProperties
  Tower column 3 : sm_lib/Body Elements/Brick Solid  GraphicAmbientColor=[0.15 0.15 0.15 1.0]  BasedOnType=Density  BrickDimensions=[T.c T.c T.h0]  BrickDimensionUnits=mm  CenterOfMass=[0 0 0]  CenterOfMassUnits=m  GraphicDiffuseColor=[0.8 0.0 0.2]  Density=1000  DensityUnits=kg/m^3  DoExposeReferenceFrame=on  GraphicEmissiveColor=[0.0 0.0 0.0 1.0]  ExportEntireGeometry=off  SerializedFrames=<Frames/>  MarkerShape=Sphere  MarkerSize=10  GraphicType=FromGeometry  InertiaType=CalculateFromGeometry  Mass=1  MassUnits=kg  MomentsOfInertia=[1 1 1]  MomentsOfInertiaUnits=kg*m^2  GraphicOpacity=0.2  ProductsOfInertia=[0 0 0]  ProductsOfInertiaUnits=kg*m^2  GraphicShininess=75  GraphicSpecularColor=[0.5 0.5 0.5 1.0]  GraphicVisPropType=SimpleVisualProperties
  Tower column 4 : sm_lib/Body Elements/Brick Solid  GraphicAmbientColor=[0.15 0.15 0.15 1.0]  BasedOnType=Density  BrickDimensions=[T.c T.c T.h0]  BrickDimensionUnits=mm  CenterOfMass=[0 0 0]  CenterOfMassUnits=m  GraphicDiffuseColor=[0.8 0.0 0.2]  Density=1000  DensityUnits=kg/m^3  DoExposeReferenceFrame=on  GraphicEmissiveColor=[0.0 0.0 0.0 1.0]  ExportEntireGeometry=off  SerializedFrames=<Frames/>  MarkerShape=Sphere  MarkerSize=10  GraphicType=FromGeometry  InertiaType=CalculateFromGeometry  Mass=1  MassUnits=kg  MomentsOfInertia=[1 1 1]  MomentsOfInertiaUnits=kg*m^2  GraphicOpacity=1.0  ProductsOfInertia=[0 0 0]  ProductsOfInertiaUnits=kg*m^2  GraphicShininess=75  GraphicSpecularColor=[0.5 0.5 0.5 1.0]  GraphicVisPropType=SimpleVisualProperties
  Tower roof1 1 : sm_lib/Body Elements/Brick Solid  GraphicAmbientColor=[0.15 0.15 0.15 1.0]  BasedOnType=Density  BrickDimensions=[T.s1 T.h1 T.hl1]  BrickDimensionUnits=mm  CenterOfMass=[0 0 0]  CenterOfMassUnits=m  GraphicDiffuseColor=[0.8 0.0 0.2]  Density=1000  DensityUnits=kg/m^3  DoExposeReferenceFrame=on  GraphicEmissiveColor=[0.0 0.0 0.0 1.0]  ExportEntireGeometry=off  SerializedFrames=<Frames/>  MarkerShape=Sphere  MarkerSize=10  GraphicType=FromGeometry  InertiaType=CalculateFromGeometry  Mass=1  MassUnits=kg  MomentsOfInertia=[1 1 1]  MomentsOfInertiaUnits=kg*m^2  GraphicOpacity=1.0  ProductsOfInertia=[0 0 0]  ProductsOfInertiaUnits=kg*m^2  GraphicShininess=75  GraphicSpecularColor=[0.5 0.5 0.5 1.0]  GraphicVisPropType=SimpleVisualProperties
  Tower roof1 2 : sm_lib/Body Elements/Brick Solid  GraphicAmbientColor=[0.15 0.15 0.15 1.0]  BasedOnType=Density  BrickDimensions=[T.s1 T.h1 T.hl1]  BrickDimensionUnits=mm  CenterOfMass=[0 0 0]  CenterOfMassUnits=m  GraphicDiffuseColor=[0.8 0.0 0.2]  Density=1000  DensityUnits=kg/m^3  DoExposeReferenceFrame=on  GraphicEmissiveColor=[0.0 0.0 0.0 1.0]  ExportEntireGeometry=off  SerializedFrames=<Frames/>  MarkerShape=Sphere  MarkerSize=10  GraphicType=FromGeometry  InertiaType=CalculateFromGeometry  Mass=1  MassUnits=kg  MomentsOfInertia=[1 1 1]  MomentsOfInertiaUnits=kg*m^2  GraphicOpacity=1.0  ProductsOfInertia=[0 0 0]  ProductsOfInertiaUnits=kg*m^2  GraphicShininess=75  GraphicSpecularColor=[0.5 0.5 0.5 1.0]  GraphicVisPropType=SimpleVisualProperties
  Tower roof1 3 : sm_lib/Body Elements/Brick Solid  GraphicAmbientColor=[0.15 0.15 0.15 1.0]  BasedOnType=Density  BrickDimensions=[T.h1 T.s1 T.hl1]  BrickDimensionUnits=mm  CenterOfMass=[0 0 0]  CenterOfMassUnits=m  GraphicDiffuseColor=[0.8 0.0 0.2]  Density=1000  DensityUnits=kg/m^3  DoExposeReferenceFrame=on  GraphicEmissiveColor=[0.0 0.0 0.0 1.0]  ExportEntireGeometry=off  SerializedFrames=<Frames/>  MarkerShape=Sphere  MarkerSize=10  GraphicType=FromGeometry  InertiaType=CalculateFromGeometry  Mass=1  MassUnits=kg  MomentsOfInertia=[1 1 1]  MomentsOfInertiaUnits=kg*m^2  GraphicOpacity=1.0  ProductsOfInertia=[0 0 0]  ProductsOfInertiaUnits=kg*m^2  GraphicShininess=75  GraphicSpecularColor=[0.5 0.5 0.5 1.0]  GraphicVisPropType=SimpleVisualProperties
  Tower roof1 4 : sm_lib/Body Elements/Brick Solid  GraphicAmbientColor=[0.15 0.15 0.15 1.0]  BasedOnType=Density  BrickDimensions=[T.h1 T.s1 T.hl1]  BrickDimensionUnits=mm  CenterOfMass=[0 0 0]  CenterOfMassUnits=m  GraphicDiffuseColor=[0.8 0.0 0.2]  Density=1000  DensityUnits=kg/m^3  DoExposeReferenceFrame=on  GraphicEmissiveColor=[0.0 0.0 0.0 1.0]  ExportEntireGeometry=off  SerializedFrames=<Frames/>  MarkerShape=Sphere  MarkerSize=10  GraphicType=FromGeometry  InertiaType=CalculateFromGeometry  Mass=1  MassUnits=kg  MomentsOfInertia=[1 1 1]  MomentsOfInertiaUnits=kg*m^2  GraphicOpacity=1.0  ProductsOfInertia=[0 0 0]  ProductsOfInertiaUnits=kg*m^2  GraphicShininess=75  GraphicSpecularColor=[0.5 0.5 0.5 1.0]  GraphicVisPropType=SimpleVisualProperties
  Tower roof1 5 : sm_lib/Body Elements/Brick Solid  GraphicAmbientColor=[0.15 0.15 0.15 1.0]  BasedOnType=Density  BrickDimensions=[T.h1 T.s1 T.hl1]  BrickDimensionUnits=mm  CenterOfMass=[0 0 0]  CenterOfMassUnits=m  GraphicDiffuseColor=[1.0 0.4 0.2]  Density=1000  DensityUnits=kg/m^3  DoExposeReferenceFrame=on  GraphicEmissiveColor=[0.0 0.0 0.0 1.0]  ExportEntireGeometry=off  SerializedFrames=<Frames/>  MarkerShape=Sphere  MarkerSize=10  GraphicType=FromGeometry  InertiaType=CalculateFromGeometry  Mass=1  MassUnits=kg  MomentsOfInertia=[1 1 1]  MomentsOfInertiaUnits=kg*m^2  GraphicOpacity=1.0  ProductsOfInertia=[0 0 0]  ProductsOfInertiaUnits=kg*m^2  GraphicShininess=75  GraphicSpecularColor=[0.5 0.5 0.5 1.0]  GraphicVisPropType=SimpleVisualProperties
  Tower roof1 6 : sm_lib/Body Elements/Brick Solid  GraphicAmbientColor=[0.15 0.15 0.15 1.0]  BasedOnType=Density  BrickDimensions=[T.h1 T.s1 T.hl1]  BrickDimensionUnits=mm  CenterOfMass=[0 0 0]  CenterOfMassUnits=m  GraphicDiffuseColor=[1.0 0.4 0.2]  Density=1000  DensityUnits=kg/m^3  DoExposeReferenceFrame=on  GraphicEmissiveColor=[0.0 0.0 0.0 1.0]  ExportEntireGeometry=off  SerializedFrames=<Frames/>  MarkerShape=Sphere  MarkerSize=10  GraphicType=FromGeometry  InertiaType=CalculateFromGeometry  Mass=1  MassUnits=kg  MomentsOfInertia=[1 1 1]  MomentsOfInertiaUnits=kg*m^2  GraphicOpacity=1.0  ProductsOfInertia=[0 0 0]  ProductsOfInertiaUnits=kg*m^2  GraphicShininess=75  GraphicSpecularColor=[0.5 0.5 0.5 1.0]  GraphicVisPropType=SimpleVisualProperties
  Tower roof2 1 : sm_lib/Body Elements/Brick Solid  GraphicAmbientColor=[0.15 0.15 0.15 1.0]  BasedOnType=Density  BrickDimensions=[T.s2 T.h2 T.hl2]  BrickDimensionUnits=mm  CenterOfMass=[0 0 0]  CenterOfMassUnits=m  GraphicDiffuseColor=[1.0 0.2 0.2]  Density=1000  DensityUnits=kg/m^3  DoExposeReferenceFrame=on  GraphicEmissiveColor=[0.0 0.0 0.0 1.0]  ExportEntireGeometry=off  SerializedFrames=<Frames/>  MarkerShape=Sphere  MarkerSize=10  GraphicType=FromGeometry  InertiaType=CalculateFromGeometry  Mass=1  MassUnits=kg  MomentsOfInertia=[1 1 1]  MomentsOfInertiaUnits=kg*m^2  GraphicOpacity=0.4  ProductsOfInertia=[0 0 0]  ProductsOfInertiaUnits=kg*m^2  GraphicShininess=75  GraphicSpecularColor=[0.5 0.5 0.5 1.0]  GraphicVisPropType=SimpleVisualProperties
  Tower roof2 2 : sm_lib/Body Elements/Brick Solid  GraphicAmbientColor=[0.15 0.15 0.15 1.0]  BasedOnType=Density  BrickDimensions=[T.s2 T.h2 T.hl2]  BrickDimensionUnits=mm  CenterOfMass=[0 0 0]  CenterOfMassUnits=m  GraphicDiffuseColor=[1.0 0.2 0.2]  Density=1000  DensityUnits=kg/m^3  DoExposeReferenceFrame=on  GraphicEmissiveColor=[0.0 0.0 0.0 1.0]  ExportEntireGeometry=off  SerializedFrames=<Frames/>  MarkerShape=Sphere  MarkerSize=10  GraphicType=FromGeometry  InertiaType=CalculateFromGeometry  Mass=1  MassUnits=kg  MomentsOfInertia=[1 1 1]  MomentsOfInertiaUnits=kg*m^2  GraphicOpacity=0.4  ProductsOfInertia=[0 0 0]  ProductsOfInertiaUnits=kg*m^2  GraphicShininess=75  GraphicSpecularColor=[0.5 0.5 0.5 1.0]  GraphicVisPropType=SimpleVisualProperties
  World : PMIOPort  Side=Left
  connections:
  Tower column 4/RConn1 -- Rigid Transform14/RConn1
  Rigid Transform17/RConn1 -- Tower roof1 3/RConn1
  Rigid Transform7/RConn1 -- Tower column 1/RConn1
  Tower roof1 2/RConn1 -- Rigid Transform16/RConn1
  Rigid Transform15/RConn1 -- Tower roof1 1/RConn1
  Rigid Transform7/LConn1 -- Rigid Transform9/LConn1 -- Rigid Transform14/LConn1 -- Rigid Transform8/LConn1 -- Rigid Transform6/LConn1 -- Rigid Transform19/LConn1 -- Rigid Transform10/LConn1 -- Rigid Transform12/LConn1 -- Rigid Transform11/LConn1 -- Rigid Transform18/LConn1 -- Rigid Transform17/LConn1 -- Rigid Transform16/LConn1 -- Rigid Transform15/LConn1 -- Rigid Transform13/RConn1
  Tower column 3/RConn1 -- Rigid Transform9/RConn1
  Tower column 2/RConn1 -- Rigid Transform8/RConn1
  Tower base/RConn1 -- Rigid Transform6/RConn1
  Rigid Transform18/RConn1 -- Tower roof1 4/RConn1
  Tower roof1 6/RConn1 -- Rigid Transform12/RConn1
  Rigid Transform11/RConn1 -- Tower roof1 5/RConn1
  Rigid Transform19/RConn1 -- Tower roof2 1/RConn1
  Rigid Transform10/RConn1 -- Tower roof2 2/RConn1
  Rigid Transform13/LConn1 -- World/RConn1

== system DemonstratorSimscape/Visualization/Sheaves Losses (Coulomb) ==
  Mux : Mux  Inputs=8
  Mux1 : Mux  Inputs=9
  Sx : Outport
  wx : Outport  Port=2
  wires:
  [S0] -> Mux/1
  [S1] -> Mux/2
  [S2] -> Mux/3
  [S3] -> Mux/4
  [S4] -> Mux/5
  [S5] -> Mux/6
  [S6] -> Mux/7
  [S7] -> Mux/8
  [w8] -> Mux1/9
  [w7] -> Mux1/8
  [w6] -> Mux1/7
  [w5] -> Mux1/6
  [w4] -> Mux1/5
  [w3] -> Mux1/4
  [w2] -> Mux1/3
  [w1] -> Mux1/2
  [w0] -> Mux1/1
  Mux/1 -> Sx/1
  Mux1/1 -> wx/1

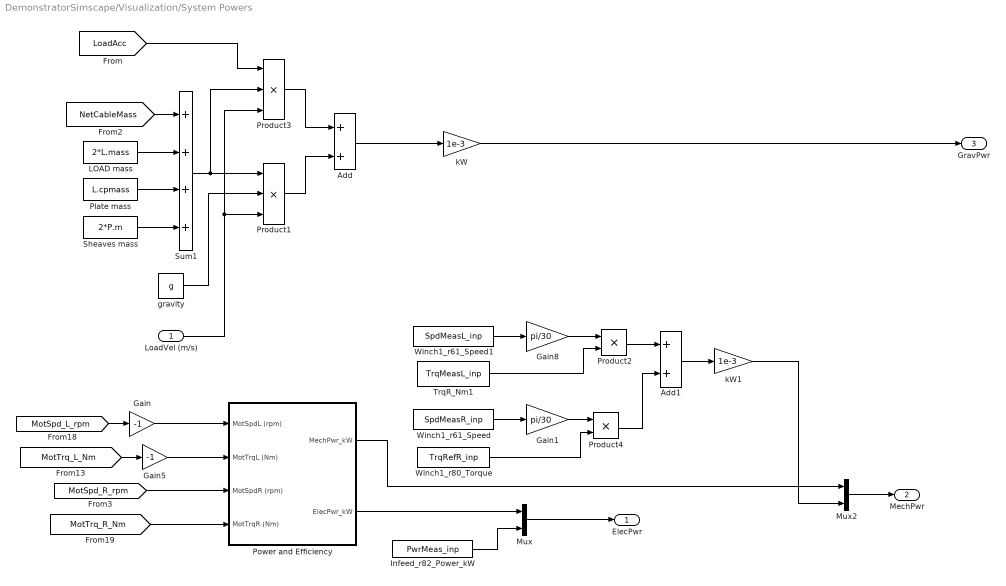
== system DemonstratorSimscape/Visualization/System Powers ==
  LoadVel (m/s) : Inport
  Add : Sum
  Add1 : Sum
  Gain : Gain  Gain=-1
  Gain1 : Gain  Gain=pi/30
  Gain5 : Gain  Gain=-1
  Gain8 : Gain  Gain=pi/30
  Infeed_r82_Power_kW : FromWorkspace  VariableName=PwrMeas_inp  Interpolate=off  OutputAfterFinalValue=Holding final value
  LOAD mass : Constant  Value=2*L.mass
  Mux : Mux  Inputs=2
  Mux2 : Mux  Inputs=2
  Plate mass : Constant  Value=L.cpmass
  Power and Efficiency : Subsystem
  Product1 : Product  Inputs=3
  Product2 : Product
  Product3 : Product  Inputs=3
  Product4 : Product
  Sheaves mass : Constant  Value=2*P.m
  Sum1 : Sum  Inputs=++++
  TrqR_Nm1 : FromWorkspace  VariableName=TrqMeasL_inp  OutputAfterFinalValue=Holding final value
  Winch1_r61_Speed : FromWorkspace  VariableName=SpdMeasR_inp  Interpolate=off  OutputAfterFinalValue=Holding final value
  Winch1_r61_Speed1 : FromWorkspace  VariableName=SpdMeasL_inp  Interpolate=off  OutputAfterFinalValue=Holding final value
  Winch1_r80_Torque : FromWorkspace  VariableName=TrqRefR_inp  Interpolate=off  OutputAfterFinalValue=Holding final value
  gravity : Constant  Value=g
  kW : Gain  Gain=1e-3
  kW1 : Gain  Gain=1e-3
  ElecPwr : Outport  VectorParamsAs1DForOutWhenUnconnected=off
  MechPwr : Outport  Port=2  VectorParamsAs1DForOutWhenUnconnected=off
  GravPwr : Outport  Port=3  VectorParamsAs1DForOutWhenUnconnected=off
  wires:
  LOAD mass/1 -> Sum1/2
  [NetCableMass] -> Sum1/1
  Plate mass/1 -> Sum1/3
  Sheaves mass/1 -> Sum1/4
  Sum1/1 -> Product3/2, Product1/1
  gravity/1 -> Product1/2
  LoadVel (m/s)/1 -> Product3/3, Product1/3
  [LoadAcc] -> Product3/1
  Product3/1 -> Add/1
  Product1/1 -> Add/2
  [MotSpd_L_rpm] -> Gain/1
  [MotTrq_L_Nm] -> Gain5/1
  Gain/1 -> Power and Efficiency/1(MotSpdL (rpm))
  Gain5/1 -> Power and Efficiency/2(MotTrqL (Nm))
  [MotTrq_R_Nm] -> Power and Efficiency/4(MotTrqR (Nm))
  [MotSpd_R_rpm] -> Power and Efficiency/3(MotSpdR (rpm))
  Infeed_r82_Power_kW/1 -> Mux/2
  Power and Efficiency/2(ElecPwr_kW) -> Mux/1
  Mux/1 -> ElecPwr/1
  kW/1 -> GravPwr/1
  Mux2/1 -> MechPwr/1
  Add/1 -> kW/1
  Winch1_r61_Speed1/1 -> Gain8/1
  Gain8/1 -> Product2/1
  TrqR_Nm1/1 -> Product2/2
  Winch1_r61_Speed/1 -> Gain1/1
  Gain1/1 -> Product4/1
  Winch1_r80_Torque/1 -> Product4/2
  Product2/1 -> Add1/1
  Product4/1 -> Add1/2
  Add1/1 -> kW1/1
  Power and Efficiency/1(MechPwr_kW) -> Mux2/1
  kW1/1 -> Mux2/2

== system DemonstratorSimscape/EM System/Drives/PLC and Drive Logic Rev3 ==
  HMI Motor 1 CSV Speed Setpoint (rpm) : Inport
  Motor 1 Actual Speed (rpm) : Inport  Port=2
  HMI Motor 1 Start Test [0...1] : Inport  Port=3
  HMI Motor 2 CSV Speed Setpoint (rpm) : Inport  Port=4
  HMI Motor 2 Start Test [0...1] : Inport  Port=5
  Motor 2 Actual Speed (rpm) : Inport  Port=6
  WAB Mode : Inport  Port=7
  WAB Motor 1 Speed_Controller Setpoint (r1438) : Inport  Port=8
  WAB Motor 2 Speed_Controller Setpoint (r1438) : Inport  Port=9
  Bus Creator : BusCreator  Inputs=2
  Bus Creator1 : BusCreator  Inputs=2
  PLC : Subsystem  TreatAsAtomicUnit=on  SystemSampleTime=Controller_sampleTime
  VFD Control1 : Subsystem  AncestorBlock=Control_Library_Rev3/VFD Control  TreatAsAtomicUnit=on  SystemSampleTime=Controller_sampleTime
  VFD Control2 : Subsystem  AncestorBlock=Control_Library_Rev3/VFD Control  TreatAsAtomicUnit=on  SystemSampleTime=Controller_sampleTime
  M1 [r0079] M_set total (Torque setpoint [Nm]) : Outport
  Winch 1 brake on command (from PLC) [0...1] : Outport  Port=2
  Motor 1 Diagnostics Bus : Outport  Port=3
  M2 [r0079] M_set total (Torque setpoint [Nm]) : Outport  Port=4
  Motor 2 Diagnostics Bus : Outport  Port=5
  Winch 2 brake on command (from PLC) [0...1] : Outport  Port=6
  wires:
  PLC/3(Motor 1 Torque limit lower (from PLC)) -> VFD Control1/4("[p1523] Torque limit lower (from PLC)")
  Motor 1 Actual Speed (rpm)/1 -> VFD Control1/1(Measured RPM)
  PLC/2(Motor 1 Torque limit upper (from PLC)) -> VFD Control1/3("[p1522] Torque limit upper (from PLC)")
  PLC/1(Motor 1 Speed Setpoint from PLC) -> VFD Control1/2("[p1070(0)] Main Setpoint (Speed setpoint from PLC)"), Bus Creator/2  "Motor 1 Speed Setpoint from PLC"
  HMI Motor 1 Start Test [0...1]/1 -> PLC/2(Motor 1 Start Test)
  VFD Control1/1("[r0079] M_set total (Torque setpoint)") -> M1 [r0079] M_set total (Torque setpoint [Nm])/1
  HMI Motor 1 CSV Speed Setpoint (rpm)/1 -> PLC/1(Motor 1 CSV Speed Setpoint)
  PLC/4(Motor 1 Droop Parameter (from PLC)) -> VFD Control1/5("[p21501] Droop Parameter from PLC")
  PLC/5(Motor 1 Enable Speed Setpoint (from PLC)) -> VFD Control1/6(Enable Speed Controller)
  VFD Control1/2(Motor 1 Diagnostics Bus) -> Bus Creator/1
  Bus Creator/1 -> Motor 1 Diagnostics Bus/1
  Bus Creator1/1 -> Motor 2 Diagnostics Bus/1
  VFD Control2/2(Motor 1 Diagnostics Bus) -> Bus Creator1/1
  VFD Control2/1("[r0079] M_set total (Torque setpoint)") -> M2 [r0079] M_set total (Torque setpoint [Nm])/1
  PLC/6(Winch 1 Brake on command (from PLC)) -> Winch 1 brake on command (from PLC) [0...1]/1
  HMI Motor 2 CSV Speed Setpoint (rpm)/1 -> PLC/3(Motor 2 CSV Speed Setpoint)
  HMI Motor 2 Start Test [0...1]/1 -> PLC/4(Motor 2 Start Test)
  Motor 2 Actual Speed (rpm)/1 -> VFD Control2/1(Measured RPM)
  PLC/7(Motor 2 Speed Setpoint from PLC) -> Bus Creator1/2, VFD Control2/2("[p1070(0)] Main Setpoint (Speed setpoint from PLC)")  "Motor 2 Speed Setpoint from PLC"
  PLC/8(Motor 2 Torque limit upper (from PLC)) -> VFD Control2/3("[p1522] Torque limit upper (from PLC)")
  PLC/9(Motor 2 Torque limit lower (from PLC)) -> VFD Control2/4("[p1523] Torque limit lower (from PLC)")
  PLC/10(Motor 2 Droop Parameter (from PLC)) -> VFD Control2/5("[p21501] Droop Parameter from PLC")
  PLC/11(Motor 2 Enable Speed Setpoint (from PLC)) -> VFD Control2/6(Enable Speed Controller)
  PLC/12(Winch 2 Brake on command (from PLC)) -> Winch 2 brake on command (from PLC) [0...1]/1
  WAB Motor 1 Speed_Controller Setpoint (r1438)/1 -> VFD Control1/8(WAB Mode Speed_Controller Setpoint (r1438))
  WAB Mode/1 -> VFD Control2/7(WAB Mode), VFD Control1/7(WAB Mode)
  WAB Motor 2 Speed_Controller Setpoint (r1438)/1 -> VFD Control2/8(WAB Mode Speed_Controller Setpoint (r1438))

== system DemonstratorSimscape/EM System/Drives/Simple Drive Model ==
  Spd_L : Inport
  SpdRef_L : Inport  Port=2
  Spd_R : Inport  Port=3
  SpdRef_R : Inport  Port=4
  Add : Sum
  Add1 : Sum
  Constant : Constant  Value=-tau_m
  Constant1 : Constant  Value=tau_m
  Gain1 : Gain  Gain=-1
  Gain3 : Gain
  LTI System : cstblocks/LTI System  sys=sysC  IC=[]
  LTI System1 : cstblocks/LTI System  sys=sysC  IC=[]
  Pwr Limits (R) : Subsystem
  Spd Limits1 : Subsystem
  Sum1 : Sum  Inputs=-+
  Sum3 : Sum  Inputs=-+
  TrqSat_L : Outport
  TrqSat_R : Outport  Port=2
  wires:
  Spd_R/1 -> Sum1/1, Pwr Limits (R)/1(Spd)
  Sum1/1 -> LTI System1/1
  SpdRef_L/1 -> Sum3/2
  Spd Limits1/1(SpdLim) -> Sum1/2
  Spd_L/1 -> Sum3/1
  Pwr Limits (R)/1(TrqSat) -> TrqSat_R/1
  SpdRef_R/1 -> Spd Limits1/1(SpdIn)
  Add/1 -> Gain3/1
  Gain3/1 -> TrqSat_L/1
  LTI System/1 -> Gain1/1
  Constant/1 -> Add/1
  Add1/1 -> Pwr Limits (R)/2(TrqIn)
  LTI System1/1 -> Add1/1
  Constant1/1 -> Add1/2
  Sum3/1 -> LTI System/1
  Gain1/1 -> Add/2
